simulink model "incompletePIDcontroller"  (R2020b)
settings: Solver=ode4  StartTime=0.0  StopTime=simulationTime  RelTol=1e-3
values from neighbouring files (symbols this model uses):
  K = 0.195    [incompletePIDcontroller.m]
  K_d = 1.0    (= 1)    [incompletePIDcontroller.m]
  K_i = 1.0    (= 1)    [incompletePIDcontroller.m]
  K_p = 1.0    (= 1)    [incompletePIDcontroller.m]
  L = 0.03    [incompletePIDcontroller.m]
  T = 0.03    [incompletePIDcontroller.m]
settings Model: Creator=Yuto  LastModifiedBy=yuto

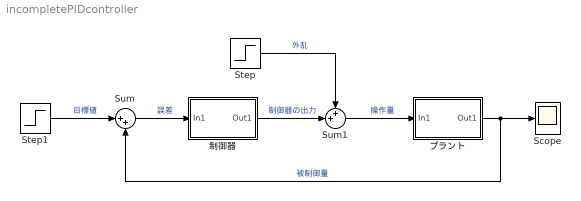
== system incompletePIDcontroller ==
  Scope : Scope
  Step : Step  SampleTime=0
  Step1 : Step  SampleTime=0
  Sum : Sum  Inputs=|++
  Sum1 : Sum  Inputs=++|
  プラント : Subsystem
  制御器 : Subsystem
  wires:
  Step1/1 -> Sum/1  "目標値"
  Step/1 -> Sum1/1  "外乱"
  Sum1/1 -> プラント/1(In1)  "操作量"
  プラント/1(Out1) -> Sum/2, Scope/1  "被制御量"
  Sum/1 -> 制御器/1(In1)  "誤差"
  制御器/1(Out1) -> Sum1/2  "制御器の出力"

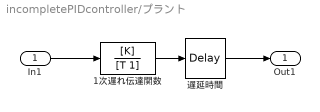
== system incompletePIDcontroller/プラント ==
  In1 : Inport
  1次遅れ伝達関数 : TransferFcn  Numerator=[K]  Denominator=[T 1]
  遅延時間 : TransportDelay  DelayTime=L
  Out1 : Outport
  wires:
  In1/1 -> 1次遅れ伝達関数/1
  1次遅れ伝達関数/1 -> 遅延時間/1
  遅延時間/1 -> Out1/1

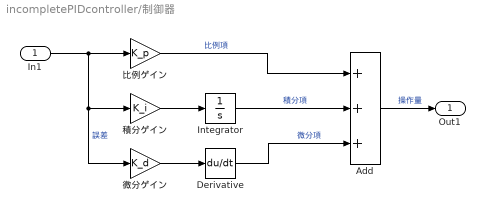
== system incompletePIDcontroller/制御器 ==
  In1 : Inport
  Add : Sum  Inputs=+++
  Derivative : Derivative
  Integrator : Integrator
  微分ゲイン : Gain  Gain=K_d
  比例ゲイン : Gain  Gain=K_p
  積分ゲイン : Gain  Gain=K_i
  Out1 : Outport
  wires:
  Add/1 -> Out1/1  "操作量"
  Derivative/1 -> Add/3  "微分項"
  積分ゲイン/1 -> Integrator/1
  Integrator/1 -> Add/2  "積分項"
  比例ゲイン/1 -> Add/1  "比例項"
  In1/1 -> 微分ゲイン/1, 積分ゲイン/1, 比例ゲイン/1  "誤差"
  微分ゲイン/1 -> Derivative/1
